simulink model "Project_Sim_Obs"  (R2025a)
settings: Solver=VariableStepAuto  StartTime=0.0  StopTime=simulation_time  RelTol=1e-3
undefined symbols (not defined in the file): N, omegaB0, pWB0, qWB0, Ts, vWB0, x0, Xref
libraries: uavutilslib x1
settings Model: Creator=franc  LastModifiedBy=franc
settings DebuggingCC: UnderspecifiedInitializationDetection=Classic  MergeDetectMultiDrivingBlocksExec=none
settings ModelReferenceCC: PropagateSignalLabelsOutOfModel=off
settings RTWCC: GPUComputeCapability=3.5

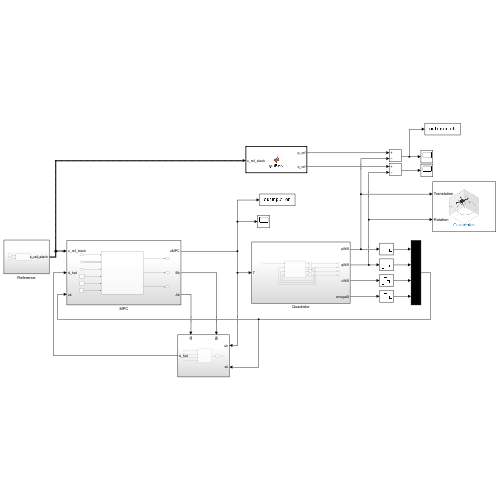
[thumbnail: Simulink's stored preview of the top-level diagram]
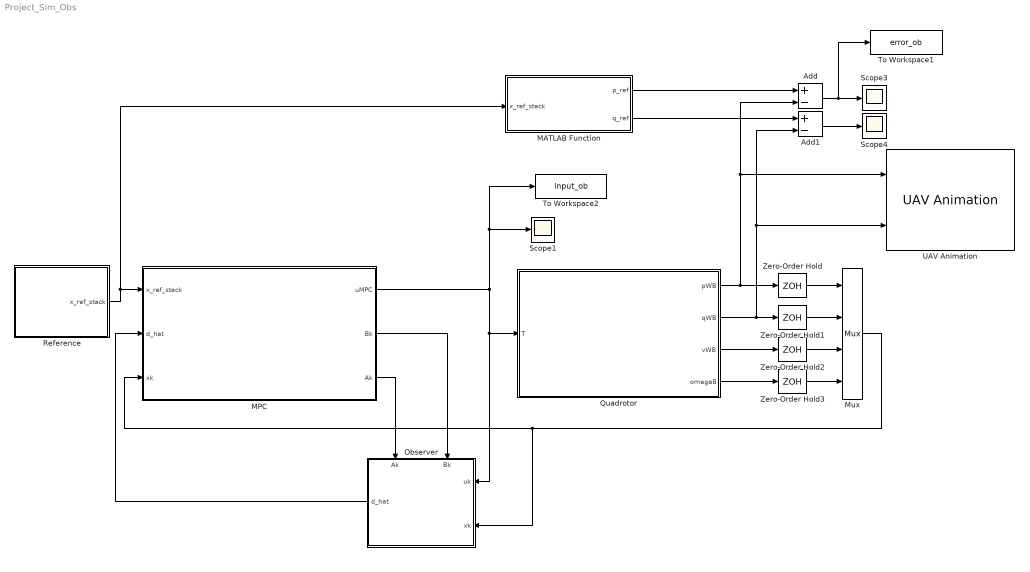
== system Project_Sim_Obs ==
  Add : Sum  Inputs=+-
  Add1 : Sum  Inputs=+-
  MATLAB Function : MATLAB Function  TreatAsAtomicUnit=on
  MPC : Subsystem
  Mux : Mux
  Observer : Subsystem
      settings: PortSchema="{\"entries\":[{\"content\":{\"sides\":[{\"content\":{\"connectorIds\":[\"In1\",\"In2\"]},\"type\":\"ConnectorPlacement.EquallySpacedRectSide\",\"uuid\":\"8d87f360-7b0e-4e82-8581-3e15549cd9b4\"},{\"content\":{\"connectorIds\":[\"Out1\"],\"side\":\"RIGHT\"},\"type\":\"ConnectorPlacement.EquallySpacedRectSide\",\"uuid\":\"74a3c6e3-6dd1-4cea-a45e-0b1089aa2f9b\"},{\"content\":{\"connectorIds\":[\"In3\",\"In4\"],\"side\":\"TOP\"},\"type\":\"ConnectorPlacement.EquallySpacedRectSide\",\"uuid\":\"e2053fa4-6f7b-463b-9a45-6bea862f2212\"}]},\"type\":\"ConnectorPlacement.EquallySpacedConnector\",\"uuid\":\"caf5610d-c963-4941-b642-2cf2cb6f8d81\"}],\"packageUris\":[\"http://schema.mathworks.com/mf0/Connector/R2020b\"],\"version\":\"1.0\"}"
  Quadrotor : Subsystem
  Reference : Subsystem
  Scope1 : Scope
      settings: ActiveDisplayYMinimum=1.5449782322617747  ActiveDisplayYMaximum=1.9488657029301115
  Scope3 : Scope
      settings: ActiveDisplayYMinimum=-0.40367061175610597  ActiveDisplayYMaximum=0.0448526765934111  DataLoggingVariableName=ScopeData4
  Scope4 : Scope
      settings: ActiveDisplayYMinimum=-0.18717400696616884  ActiveDisplayYMaximum=0.18977772043834604  DataLoggingVariableName=ScopeData5
  To Workspace1 : ToWorkspace  VariableName=error_ob  SaveFormat=Structure With Time  SampleTime=-1
  To Workspace2 : ToWorkspace  VariableName=input_ob  SaveFormat=Structure With Time  SampleTime=-1
  UAV Animation : uavutilslib/UAV Animation  NumUAV=1  DynamicUAVConfig=off  UAVType=Multirotor  UAVSize=1  UAVColor=[1 0 0]  UAVTrajectoryAlpha=1  InertialZDirection=Up  RotationFormat=Quaternion  DrawMarkers=off  SampleTime=-1
  Zero-Order Hold{,1..3} (4 alike) : ZeroOrderHold  SampleTime=Ts
  wires:
  Quadrotor/1(pWB) -> UAV Animation/1, Add/2, Zero-Order Hold/1
  Quadrotor/2(qWB) -> UAV Animation/2, Add1/2, Zero-Order Hold1/1
  Quadrotor/3(vWB) -> Zero-Order Hold2/1
  Quadrotor/4(omegaB) -> Zero-Order Hold3/1
  Zero-Order Hold3/1 -> Mux/4
  Zero-Order Hold2/1 -> Mux/3
  Zero-Order Hold1/1 -> Mux/2
  Zero-Order Hold/1 -> Mux/1
  Mux/1 -> Observer/2(xk), MPC/3(xk)
  Reference/1(x_ref_stack) -> MATLAB Function/1(x_ref_stack), MPC/1(x_ref_stack)
  MATLAB Function/1(p_ref) -> Add/1
  Add/1 -> To Workspace1/1, Scope3/1
  MATLAB Function/2(q_ref) -> Add1/1
  Add1/1 -> Scope4/1
  MPC/1(uMPC) -> Observer/1(uk), Quadrotor/1(T), To Workspace2/1, Scope1/1
  MPC/2(Bk) -> Observer/3(Bk)
  MPC/3(Ak) -> Observer/4(Ak)
  Observer/1(d_hat) -> MPC/2(d_hat)

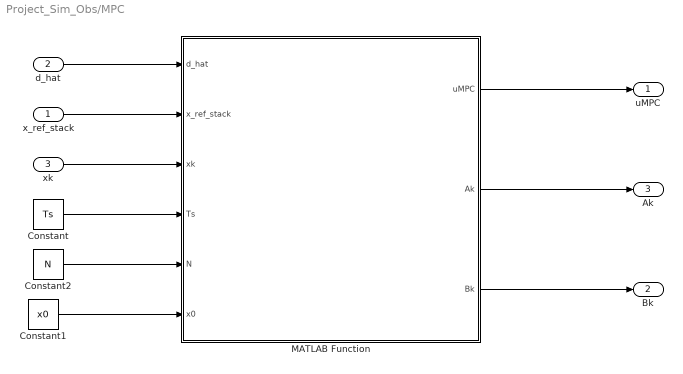
== system Project_Sim_Obs/MPC ==
  x_ref_stack : Inport
  d_hat : Inport  Port=2
  xk : Inport  Port=3
  Constant : Constant  Value=Ts
  Constant1 : Constant  Value=x0
  Constant2 : Constant  Value=N
  MATLAB Function : MATLAB Function  TreatAsAtomicUnit=on
  uMPC : Outport
  Bk : Outport  Port=2
  Ak : Outport  Port=3
  wires:
  Constant/1 -> MATLAB Function/4(Ts)
  Constant1/1 -> MATLAB Function/6(x0)
  xk/1 -> MATLAB Function/3(xk)
  MATLAB Function/1(uMPC) -> uMPC/1
  Constant2/1 -> MATLAB Function/5(N)
  x_ref_stack/1 -> MATLAB Function/2(x_ref_stack)
  MATLAB Function/2(Ak) -> Ak/1
  MATLAB Function/3(Bk) -> Bk/1
  d_hat/1 -> MATLAB Function/1(d_hat)

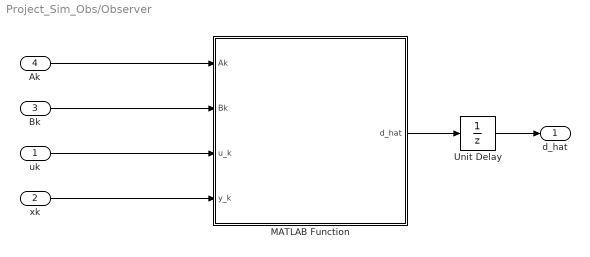
== system Project_Sim_Obs/Observer ==
  uk : Inport
  xk : Inport  Port=2
  Bk : Inport  Port=3
  Ak : Inport  Port=4
  MATLAB Function : MATLAB Function  TreatAsAtomicUnit=on
  Unit Delay : UnitDelay  SampleTime=-1  HasFrameUpgradeWarning=on
  d_hat : Outport
  wires:
  Ak/1 -> MATLAB Function/1(Ak)
  Bk/1 -> MATLAB Function/2(Bk)
  uk/1 -> MATLAB Function/3(u_k)
  xk/1 -> MATLAB Function/4(y_k)
  MATLAB Function/1(d_hat) -> Unit Delay/1
  Unit Delay/1 -> d_hat/1

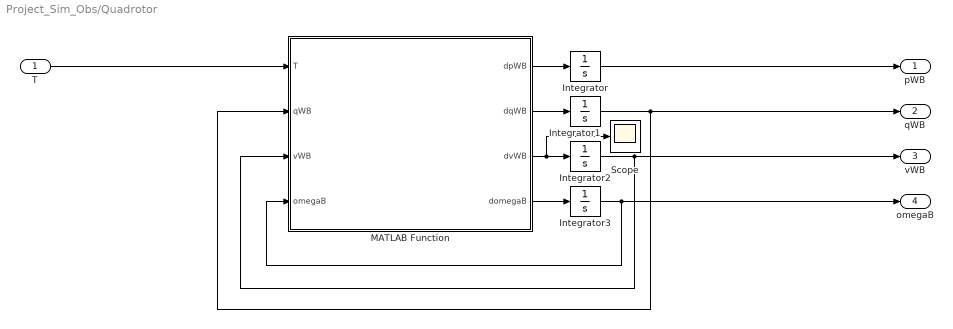
== system Project_Sim_Obs/Quadrotor ==
  T : Inport
  Integrator : Integrator  InitialCondition=pWB0
  Integrator1 : Integrator  InitialCondition=qWB0
  Integrator2 : Integrator  InitialCondition=vWB0
  Integrator3 : Integrator  InitialCondition=omegaB0
  MATLAB Function : MATLAB Function  TreatAsAtomicUnit=on
  Scope : Scope
      settings: ActiveDisplayYMinimum=-10.516652542372883  ActiveDisplayYMaximum=1.7458474576271188  DataLoggingVariableName=ScopeData2
  pWB : Outport
  qWB : Outport  Port=2
  vWB : Outport  Port=3
  omegaB : Outport  Port=4
  wires:
  T/1 -> MATLAB Function/1(T)
  MATLAB Function/1(dpWB) -> Integrator/1
  MATLAB Function/2(dqWB) -> Integrator1/1
  MATLAB Function/3(dvWB) -> Scope/1, Integrator2/1
  MATLAB Function/4(domegaB) -> Integrator3/1
  Integrator1/1 -> MATLAB Function/2(qWB), qWB/1
  Integrator2/1 -> MATLAB Function/3(vWB), vWB/1
  Integrator3/1 -> MATLAB Function/4(omegaB), omegaB/1
  Integrator/1 -> pWB/1

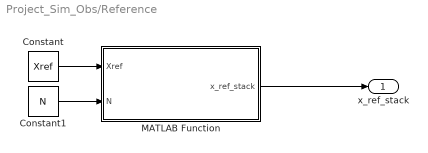
== system Project_Sim_Obs/Reference ==
  Constant : Constant  Value=Xref
  Constant1 : Constant  Value=N
  MATLAB Function : MATLAB Function  TreatAsAtomicUnit=on  SystemSampleTime=Ts
  x_ref_stack : Outport
  wires:
  Constant1/1 -> MATLAB Function/2(N)
  Constant/1 -> MATLAB Function/1(Xref)
  MATLAB Function/1(x_ref_stack) -> x_ref_stack/1

== matlab function Project_Sim_Obs/MPC/MATLAB Function ==
  data: d_hat input size=2; x_ref_stack input; xk input size=13; uMPC output size=4; Ts input size=1; N input; x0 input size=13; Ak output; Bk output
function [uMPC, Ak, Bk] = MPC(d_hat, x_ref_stack,xk,Ts,N,x0)

% Initialization
persistent ubar x0_guess u0_guess;

u_hover = 0.716*9.81/4; 
if isempty(ubar)
    ubar = u_hover*ones(4,1);
end

% Dimensions
nx = 13;
nu = 4;

% Cost parameters
R = 10*eye(nu);
Q = diag(400*[10 10 200 1 1 1 1 1 1 1 1 1 1]);

% Inequality constraints per time step (input) (H_u*u <= k_u)
rpm_max = 10880;
omega_max = rpm_max*2*pi/60;
u_max = 1.6e-2*omega_max^2;

H_u = [ eye(nu);
      -eye(nu)];
k_u = [ u_max*ones(nu,1);
       zeros(nu,1)];

% Inequality constraints per time step (state, fictional) (H_x*x <= k_x)
x_min = -1e6*ones(nx,1);
x_max = 1e6*ones(nx,1);
H_x = [ eye(nx);
       -eye(nx)];
k_x = [ x_max;
       -x_min ];

% System dynamics (Computation of the linearized system around the current state)
[Ak,Bk,ck] = lin_fdyn_central(xk, ubar, Ts);

% Inequality constraints for the whole horizon (A*z <= b)
% z = [x0,x1,...,xN-1,xN,u0,u1,...,uN-1]'
Ax = kron(eye(N+1), H_x);
bx = repmat(k_x, N+1, 1);
Au = kron(eye(N), H_u);
bu = repmat(k_u, N, 1);

A = blkdiag(Ax,Au);
b = [bx;bu];

% Equality constraints
Aeq=zeros(nx*(N+1),nx*(N+1)+nu*N);
beq=zeros(nx*(N+1),1);

% Disturb Matrices
nd = 2;
Bd = [eye(nd); zeros(nx-nd,nd)];
Cd = [eye(nd); zeros(nx-nd,nd)];

for k=0:N-1 % Linearized system dynamics constraints 
    Aeq(nx*k+1:nx*(k+1),1:nx*(N+1))=[zeros(nx,nx*k),Ak,-eye(nx),zeros(nx,nx*(N-1-k))];
    Aeq(nx*k+1:nx*(k+1),nx*(N+1)+1:end)=[zeros(nx,nu*k),Bk,zeros(nx,nu*(N-1-k))];
    beq(nx*k+1:nx*(k+1)) = -ck-Bd*d_hat;
end

% Initial condition constraints
Aeq(nx*N+1:nx*(N+1),:)=[eye(nx),zeros(nx,nu*N+nx*N)];
beq(nx*N+1:nx*(N+1))=xk;

% Cost function
Qstack = kron(eye(N+1), Q); % Q, but for the whole horizon
Rstack = kron(eye(N), R); % R, but for the whole horizon
    
HQP = blkdiag(Qstack,Rstack); % Overall cost

% Observer action
C  = eye(nx);
r_t = x_ref_stack(1:nx);
M = [Ak-eye(nx), Bk;
     C, zeros(nx,nu)];
rhs = [-Bd*d_hat;
       r_t-Cd*d_hat];
sol = M\rhs;
u_ss = sol(nx+1:nx+nu);

u_ref_stack = repmat(u_ss, N, 1); % Reference on the input retrieved from the observer action
fQP = -HQP * [x_ref_stack; u_ref_stack]; % x and u centered on their references

% solver parameters
if isempty(x0_guess)
    x0_guess = repmat(x0,N+1,1);
end
if isempty(u0_guess)
    u0_guess = repmat(u_hover*ones(nu,1),N,1);
end
tol_opt       = 1e-8;
options = optimoptions('quadprog', ...
                       'Algorithm', 'active-set', ...
                       'MaxIterations', 10000, ...
                       'OptimalityTolerance', tol_opt, ...
                       'StepTolerance', tol_opt);

% optimization
solutionOL = quadprog(HQP,fQP,A,b,Aeq,beq,[],[],[x0_guess;u0_guess],options);

% Derive the optimal predicted state and input sequence
x_OL_tilde = solutionOL(1:nx*(N+1),1);
u_OL_tilde = solutionOL(nx*(N+1)+1:end,1);
x_OL = reshape(x_OL_tilde,nx,N+1);
u_OL = reshape(u_OL_tilde,nu,N);

% Prepare warmstart solution for next time step 
x0_guess = [x_OL_tilde(nx+1:end);zeros(nx,1)];
u0_guess = [u_OL_tilde(nu+1:end);zeros(nu,1)];

% Imposing MPC action
uMPC = u_OL(:,1);
ubar = uMPC;

%% functions for system dynamics

    function [Ak,Bk,ck] = lin_fdyn_central(xbar, ubar, dt) % system dynamics linearization

        % Retrieving the Nonlinear system dynamics
        nnx = numel(xbar);
        nnu = numel(ubar);
        f0 = fRK4(xbar, ubar, dt);

        % denominator settings
        hx = (eps^(1/3))*max(1, abs(xbar));
        hu = (eps^(1/3))*max(1, abs(ubar));

        % Matrices initialization
        Ak = zeros(nnx);
        Bk = zeros(nnx,nnu);

        for i = 1:nnx % Ak computation
            dx = zeros(nnx,1);
            dx(i) = hx(i);
            fp = fRK4(xbar+dx, ubar, dt);
            fm = fRK4(xbar-dx, ubar, dt);
            Ak(:,i) = (fp-fm)/(2*hx(i));
        end

        for j = 1:nnu % Bk computation
            du = zeros(nnu,1);
            du(j) = hu(j);
            fp = fRK4(xbar, ubar+du, dt);
            fm = fRK4(xbar, ubar-du, dt);
            Bk(:,j) = (fp-fm)/(2*hu(j));
       end

       ck = f0 - Ak*xbar - Bk*ubar; % Residual computation
    end


    function xk1 = fRK4(xk,uk,deltaT) % Runge-Kutta 4th order discretization
        k1 = f(xk,uk);
        k2 = f(xk+deltaT/2*k1,uk);
        k3 = f(xk+deltaT/2*k2,uk);
        k4 = f(xk+deltaT*k3,uk);
        xk1 = xk+deltaT/6*(k1+2*k2+2*k3+k4);
    end

    function dotx = f(x,u) % Nonlinear Nominal system dynamics (see Plant code for details)
    g = 9.81;
    g_vec = [0 0 -g]';

    T0 = u(1);
    T1 = u(2);
    T2 = u(3);
    T3 = u(4);

    TB = [0 0 T0+T1+T2+T3]';
    m = 0.716;
    
    Jx = 0.007;
    Jy = Jx;
    Jz = 0.012;

    J = diag([Jx,Jy,Jz]);

    xx = zeros(4,1);
    yy = zeros(4,1);
    dxx = zeros(4,1);
    dyy = zeros(4,1);

    l = 0.17;
    theta = [0 pi/2 pi -pi/2]';
    for i=1:4
       xx(i)=l*cos(theta(i));
       yy(i)=l*sin(theta(i));
    end
    for i=1:4
        dxx(i)=abs(yy(i));
        dyy(i)=abs(xx(i));
    end
    cT = 1.6e-2;
    P = [-dxx(1) -dxx(2) dxx(3) dxx(4);
         dyy(1) -dyy(2) -dyy(3) dyy(4)
         -cT     cT    -cT    cT];

    tauB = P*[T0 T1 T2 T3]';

    pWB = x(1:3);
    qWB = x(4:7);
    vWB = x(8:10);
    omegaB = x(11:13);

    dpWB = vWB;
    dqWB = quatmultiply(qWB,[0 omegaB'/2]');
    dvWB = quaternion_product(qWB,TB/m)+g_vec;
    domegaB = inv(J)*(tauB - cross(omegaB, J*omegaB));

    dotx = [dpWB;dqWB;dvWB;domegaB];


    function res = quaternion_product(q, vec) % quaternion * vector
        q = q/ norm(q);
        q_conj = [q(1) -q(2) -q(3) -q(4)]';
        q_vec = [0 vec']';
        res = quatmultiply(q, q_vec);
        res = quatmultiply(res,q_conj);
        res = res(2:4);
    end


    function q_out = quatmultiply(q1, q2) % quaternion multiplication

    qw1 = q1(1); qx1 = q1(2); qy1 = q1(3); qz1 = q1(4);
    qw2 = q2(1); qx2 = q2(2); qy2 = q2(3); qz2 = q2(4);

    q_out = [qw1*qw2 - qx1*qx2 - qy1*qy2 - qz1*qz2;
             qw1*qx2 + qx1*qw2 + qy1*qz2 - qz1*qy2; 
             qw1*qy2 - qx1*qz2 + qy1*qw2 + qz1*qx2; 
             qw1*qz2 + qx1*qy2 - qy1*qx2 + qz1*qw2];
    end
    end
end

== matlab function Project_Sim_Obs/Quadrotor/MATLAB Function ==
  data: T input size=4; qWB input size=4; vWB input size=3; dpWB output size=3; dqWB output size=4; dvWB output size=3; domegaB output size=3; omegaB input size=3
function [dpWB,dqWB,dvWB,domegaB] = dynamics(T,qWB,vWB,omegaB)

    % gravity term
    g = 9.81;
    g_vec = [0 0 -g]';

    % thrusts
    T0 = T(1);
    T1 = T(2);
    T2 = T(3);
    T3 = T(4);
    TB = [0 0 T0+T1+T2+T3]';

    % mass
    m = 0.716;
    
    % Inertia
    Jx = 0.007;
    Jy = Jx;
    Jz = 0.012;
    J = diag([Jx,Jy,Jz]);

    % Allocation Matrix computation
    l = 0.17;
    theta = [0 pi/2 pi -pi/2]';
    xx = zeros(4,1);
    yy = zeros(4,1);
    dxx = zeros(4,1);
    dyy = zeros(4,1);
    for i=1:4
       xx(i)=l*cos(theta(i));
       yy(i)=l*sin(theta(i));
    end
    for i=1:4
        dxx(i)=abs(yy(i));
        dyy(i)=abs(xx(i));
    end
    cT = 1.6e-2;
    P = [-dxx(1) -dxx(2) dxx(3) dxx(4);
         dyy(1) -dyy(2) -dyy(3) dyy(4)
         -cT     cT    -cT    cT];

    tauB = P*[T0 T1 T2 T3]';

    % wind effect
    v_wind = [1 1 0]';

    % model dynamics
    dpWB = vWB+v_wind;
    dqWB = quatmultiply(qWB,[0 omegaB'/2]');
    dvWB = quaternion_product(qWB,TB/m)+g_vec;
    domegaB = inv(J)*(tauB - cross(omegaB, J*omegaB));


    function res = quaternion_product(q, vec) % quaternion * vector
        q = q/ norm(q);
        q_conj = [q(1) -q(2) -q(3) -q(4)]';
        q_vec = [0 vec']';
        tmp_1 = quatmultiply(q, q_vec);
        tmp_2 = quatmultiply(tmp_1,q_conj);
        res = tmp_2(2:4);
    end


    function q_out = quatmultiply(q1, q2) % quaternion product

    qw1 = q1(1); qx1 = q1(2); qy1 = q1(3); qz1 = q1(4);
    qw2 = q2(1); qx2 = q2(2); qy2 = q2(3); qz2 = q2(4);

    q_out = [qw1*qw2 - qx1*qx2 - qy1*qy2 - qz1*qz2; 
             qw1*qx2 + qx1*qw2 + qy1*qz2 - qz1*qy2; 
             qw1*qy2 - qx1*qz2 + qy1*qw2 + qz1*qx2; 
             qw1*qz2 + qx1*qy2 - qy1*qx2 + qz1*qw2];
    end

end

== matlab function Project_Sim_Obs/Reference/MATLAB Function ==
  data: Xref input; x_ref_stack output size=[13*(N+1), 1]; N input
function x_ref_stack = buildRefStack(Xref, N)

% This code simply retrieves the whole trajectory and gives as output the
% trajectory between current time and the end of the horizon for the MPC

    persistent k;
    if isempty(k)
        k = 1;
    end

    nx = 13;
    Ttot = size(Xref, 2);
    k_end = k + N;
    if k_end > Ttot
        k_end = Ttot;
    end

    Xslice = Xref(:, k:k_end);
    missing = (N+1) - size(Xslice,2);
    if missing > 0
        lastcol = Xslice(:, end);
        Xslice = [Xslice, repmat(lastcol, 1, missing)];
    end
    x_ref_stack = reshape(Xslice, nx*(N+1), 1);

    if k < Ttot
        k = k + 1;
    end
end

== matlab function Project_Sim_Obs/MATLAB Function ==
  data: x_ref_stack input; p_ref output; q_ref output
function [p_ref,q_ref] = getRefs(x_ref_stack)
    p_ref = x_ref_stack(1:3);
    q_ref = x_ref_stack(4:7);
end

== matlab function Project_Sim_Obs/Observer/MATLAB Function ==
  data: Ak input size=[13 13]; Bk input size=[13 4]; u_k input size=4; y_k input size=13; d_hat output size=2
function d_hat = offsetFreeObserver(Ak, Bk, u_k, y_k)

    % dimensions
    nx = size(Ak,1);
    nu = size(Bk,2);
    nd = 2;

    persistent z_hat
    if isempty(z_hat)
        z_hat = zeros(nx+nd,1);
    end

    % Disturb Matrices
    Bd = [eye(nd); zeros(nx-nd,nd)];
    C  = eye(nx);
    Cd = [eye(nd); zeros(nx-nd,nd)];

    % Augmented Matrices
    A_e = [Ak, Bd; zeros(nd,nx), eye(nd)];
    B_e = [Bk; zeros(nd,nu)];
    C_e = [C, Cd];

    % Observation Matrices
    L_x = 0.5*eye(nx);
    L_d = 0.5*[eye(nd), zeros(nd,nx-nd)];
    L_e = [L_x; L_d];

    % Observer dynamics
    y_hat = C_e * z_hat;
    err = y_hat - y_k;
    z_hat = A_e*z_hat+B_e*u_k-L_e*err;

    % Retrieving the disturbance
    d_hat = z_hat(nx+1:end);
end
